simulink model "Controllo_LQG_int"  (R2023b)
settings: Solver=ode45  StartTime=0.0  StopTime=20  MaxStep=0.005  RelTol=1e-3  EnableMultiTasking=on
undefined symbols (not defined in the file): A, B, C, C_add, D, KF, Kint1, Kint2, Qt, Rt
libraries: simulink x2
settings Model: Creator=roberto  LastModifiedBy=roberto_ambrosino
settings SolverCC: AlgebraicLoopSolver=TrustRegion
settings DataIOCC: LimitDataPoints=on  SaveFormat=Array  ReturnWorkspaceOutputs=off
settings OptimizationCC: LifeSpan=inf
settings DebuggingCC: UnconnectedInputMsg=warning  UnconnectedOutputMsg=warning  UnconnectedLineMsg=warning  SFUnexpectedBacktrackingDiag=warning  SFNoUnconditionalDefaultTransitionDiag=warning  SFExecutionAtInitializationDiag=none  ArithmeticOperatorsInVariantConditions=warning
settings HardwareCC: ProdBitPerPointer=32  ProdBitPerSizeT=32  ProdBitPerPtrDiffT=32  ProdLargestAtomicFloat=None  ProdIntDivRoundTo=Undefined  ProdEndianess=Unspecified  ProdWordSize=32  ProdHWDeviceType=32-bit Generic
settings ModelReferenceCC: EnableRefExpFcnMdlSchedulingChecks=on  PropagateSignalLabelsOutOfModel=off
settings SFSimCC: SimUseLocalCustomCode=off  CustomCodeUndefinedFunction=UseInterfaceOnly
settings RTWCC: RTWUseLocalCustomCode=off  DLArmComputeVersion=19.05
settings CodeAppCC: StateflowObjectComments=on
settings GRTTargetCC: TargetLangStandard=C89/C90 (ANSI)
settings ConfigComp: CovMetricSettings=dw  CovSaveCumulativeToWorkspaceVar=on  CovSaveSingleToWorkspaceVar=on  CovExternalEMLEnable=off

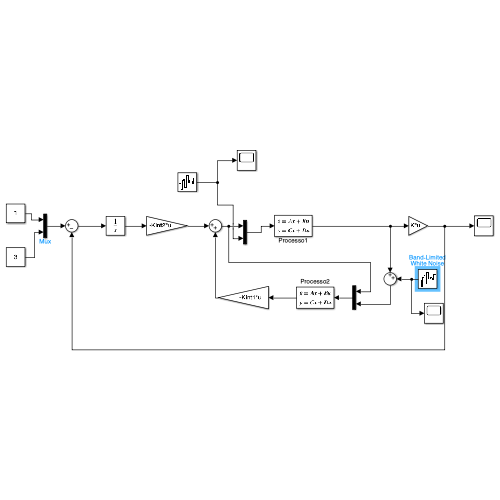
[thumbnail: Simulink's stored preview of the top-level diagram]
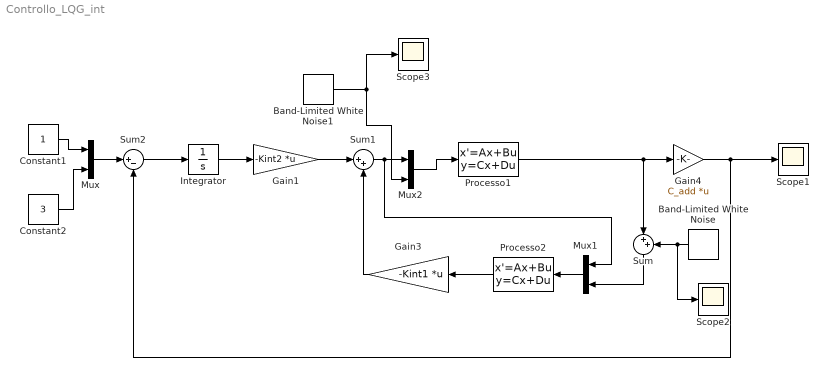
== system Controllo_LQG_int ==
  Band-Limited White Noise : simulink/Sources/Band-Limited White Noise  Cov=diag(Rt)  Ts=0.01  seed=[23341]
  Band-Limited White Noise1 : simulink/Sources/Band-Limited White Noise  Cov=diag(Qt)  Ts=0.01  seed=[23341]
  Constant1 : Constant
  Constant2 : Constant  Value=3
  Gain1 : Gain  Gain=-Kint2  Multiplication=Matrix(K*u)
  Gain3 : Gain  Gain=-Kint1  Multiplication=Matrix(K*u)
  Gain4 : Gain  Gain=C_add  Multiplication=Matrix(K*u)
  Integrator : Integrator
  Mux : Mux  Inputs=2
  Mux1 : Mux  Inputs=2
  Mux2 : Mux  Inputs=[2 6]
  Processo1 : StateSpace  A=A  B=[B eye(6)]  C=C  D=[D zeros(size(C,1),6)]  InitialCondition=[1 0 2 0 3 0]
  Processo2 : StateSpace  A=KF.A  B=KF.B  C=KF.C  D=KF.D  InitialCondition=[1 0 2 0 3 0]
  Scope1 : Scope
  Scope2 : Scope
  Scope3 : Scope
  Sum : Sum  Inputs=|++
  Sum1 : Sum  Inputs=|++
  Sum2 : Sum  Inputs=|+-
  wires:
  Processo1/1 -> Sum/1, Gain4/1
  Gain4/1 -> Sum2/2, Scope1/1
  Gain3/1 -> Sum1/2
  Sum2/1 -> Integrator/1
  Integrator/1 -> Gain1/1
  Gain1/1 -> Sum1/1
  Mux/1 -> Sum2/1
  Constant1/1 -> Mux/1
  Constant2/1 -> Mux/2
  Mux1/1 -> Processo2/1
  Processo2/1 -> Gain3/1
  Band-Limited White Noise/1 -> Scope2/1, Sum/2
  Sum/1 -> Mux1/2
  Mux2/1 -> Processo1/1
  Sum1/1 -> Mux1/1, Mux2/1
  Band-Limited White Noise1/1 -> Mux2/2, Scope3/1
